simulink model "projectTest_R2013a_2"  (Simulink 9.2)
settings: Solver=ode45  StartTime=0.0  StopTime=3*times(end)  RelTol=1e-3  EnableMultiTasking=on
values from neighbouring files (symbols this model uses):
  Noise = 0    [student_test.m]
libraries: cstblocks x2, simulink x1
settings Model: Creator=trevorashley  LastModifiedBy=sean
settings DataIOCC: SignalLoggingSaveFormat=Dataset
settings DebuggingCC: SolverPrmCheckMsg=warning  FcnCallInpInsideContextMsg=error
settings GRTTargetCC: CombineOutputUpdateFcns=on  GRTInterface=off
settings ConfigComp: CovSFcnEnable=off

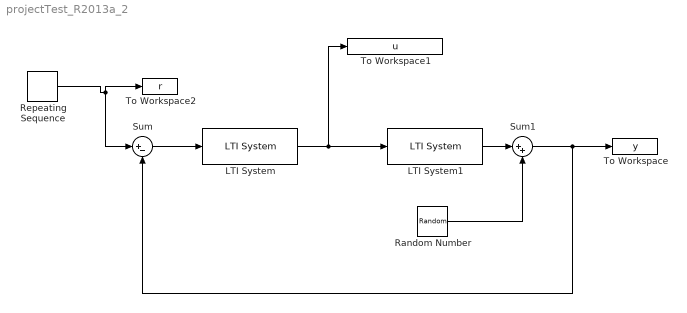
== system projectTest_R2013a_2 ==
  LTI System : cstblocks/LTI System  sys=D_c  IC=[]
  LTI System1 : cstblocks/LTI System  sys=G_nom  IC=[]
  Random Number : RandomNumber  Variance=Noise  SampleTime=0
  Repeating Sequence : simulink/Sources/Repeating Sequence  rep_seq_t=times  rep_seq_y=outputVals
  Sum : Sum  Inputs=|+-
  Sum1 : Sum  Inputs=|++
  To Workspace : ToWorkspace  VariableName=y  SaveFormat=Timeseries  SampleTime=-1
  To Workspace1 : ToWorkspace  VariableName=u  SaveFormat=Timeseries  SampleTime=-1
  To Workspace2 : ToWorkspace  VariableName=r  SaveFormat=Timeseries  SampleTime=-1
  wires:
  Sum/1 -> LTI System/1
  LTI System/1 -> To Workspace1/1, LTI System1/1
  LTI System1/1 -> Sum1/1
  Sum1/1 -> To Workspace/1, Sum/2
  Repeating Sequence/1 -> To Workspace2/1, Sum/1
  Random Number/1 -> Sum1/2
